simulink model "AmpelkreuzungV4_7"  (R2024b)
settings: Solver=FixedStepAuto  StartTime=0.0  StopTime=450  FixedStep=1  RelTol=1e-3
model workspace (MATLAB code in the model file):
  | function [autos_l1, autos_rg1, autos_2l, autos_2rg, autos_3l, autos_3rg, autos_4, fehler] = generateCars(Auslastung)
  |     if (auslastung == 1)
  |         autos_l1 = round(randn());
  |         autos_rg1 = round(randn());
  |         autos_2l = round(randn());
  |         autos_2rg = round(randn());
  |         autos_3l = round(randn());
  |         autos_3rg = round(randn());
  |         autos_4 = round(randn());
  |     else
  |         fehler = 1;
  |     end
  | 
  |     if (auslastung == 2)
  |         autos_l1 = round(randn());
  |         autos_rg1 = round(4 + 2 * randn());
  |         autos_2l = round(1 + randn());
  |         autos_2rg = round(4 + 2 * randn());
  |         autos_3l = round(randn());
  |         autos_3rg = round(2 + randn());
  |         autos_4 = round(1 + randn());
  |     else
  |         fehler = 1;
  |     end
  | 
  |     if (auslastung == 3)
  |         autos_l1 = round(1.5 + randn());
  |         autos_rg1 = round(7 + 2 * randn());
  |         autos_2l = round(2 + randn());
  |         autos_2rg = round(7 + 2 * randn());
  |         autos_3l = round(2 * randn());
  |         autos_3rg = round(3 + randn());
  |         autos_4 = round(2 + randn());
  |     else
  |         fehler = 1;
  |     end
  | 
  |     if (auslastung == 4)
  |         autos_l1 = round(2.5 + randn());
  |         autos_rg1 = round(13 + 3 * randn());
  |         autos_2l = round(5 + randn());
  |         autos_2rg = round(13 + 3 * randn());
  |         autos_3l = round(2 + randn());
  |         autos_3rg = round(2 + randn());
  |         autos_4 = round(5 + randn());
  |     else
  |         fehler = 1;
  |     end
  | end
(part 2 of 2)

== stateflow chart AmpelkreuzungV4_7/Chart ==
  state Start
    entry:
    rot1_l = 1;
    gelb1_l = 0;
    gruen1_l = 0;
    rot1_rg = 1;
    gelb1_rg = 0;
    gruen1_rg = 0;
    rot2 = 1;
    gelb2 = 0;
    gruen2 = 0;
    rot3_l = 1;
    gelb3_l = 0;
    gruen3_l = 0;
    rot3_rg = 1;
    gelb3_rg = 0;
    gruen3_rg = 0;
    rot4 = 1;
    gelb4 = 0;
    gruen4 = 0;
    rot5 = 1;
    gruen5 = 0;
    rot6 = 1;
    gruen6 = 0;
    rot7 = 1;
    gruen7 = 0;
    rot8 = 1;
    gruen8 = 0;
    timeCounter = 0;
    timer_spuren = [0 0 0 0 0 0 0];
    gesamtZeit = 0;
    %alle_autos = [0 0 0 0 0 0 0; 0 0 0 0 0 0 0];
    spur1 = zeros(1,N/2);
    spur2 = zeros(1,N/2);
    spur3 = zeros(1,N/2);
    spur4 = zeros(1,N/2);
    spur5 = zeros(1,N/2);
    spur6 = zeros(1,N/2);
    spur7 = zeros(1,N/2);
    autos_auf_spur1 = 0;
    autos_auf_spur2 = 0;
    autos_auf_spur3 = 0;
    autos_auf_spur4 = 0;
    autos_auf_spur5 = 0;
    autos_auf_spur6 = 0;
    autos_auf_spur7 = 0;
    counter = [0 0 0 0 0 0 0];
    anz_autos1 = 0;
    anz_autos2 = 0;
    anz_autos3 = 0;
    anz_autos4 = 0;
    anz_autos5 = 0;
    anz_autos6 = 0;
    anz_autos7 = 0;
    wartezeit_spur1_ges = 0;
    wartezeit_spur2_ges = 0;
    wartezeit_spur3_ges = 0;
    wartezeit_spur4_ges = 0;
    wartezeit_spur5_ges = 0;
    wartezeit_spur6_ges = 0;
    wartezeit_spur7_ges = 0;
  state dokumentiere_startzeiten_initialisiere_wartezeiten
    en:
    startzeiten1 = spur1;
    startzeiten2 = spur2;
    startzeiten3 = spur3;
    startzeiten4 = spur4;
    startzeiten5 = spur5;
    startzeiten6 = spur6;
    startzeiten7 = spur7;
    wartezeiten1 = zeros(1, length(startzeiten1));
    wartezeiten2 = zeros(1, length(startzeiten2));
    wartezeiten3 = zeros(1, length(startzeiten3));
    wartezeiten4 = zeros(1, length(startzeiten4));
    wartezeiten5 = zeros(1, length(startzeiten5));
    wartezeiten6 = zeros(1, length(startzeiten6));
    wartezeiten7 = zeros(1, length(startzeiten7));
  state endzeiten_initialisieren
    en:
    endzeiten1 = zeros(1, length(spur1));
    endzeiten2 = zeros(1, length(spur2));
    endzeiten3 = zeros(1, length(spur3));
    endzeiten4 = zeros(1, length(spur4));
    endzeiten5 = zeros(1, length(spur5));
    endzeiten6 = zeros(1, length(spur6));
    endzeiten7 = zeros(1, length(spur7));
  state rg1_ampel2_rotgelb
    entry:
    gelb1_rg = 1;
    gelb2 = 1;
  state l1_rg1_rotgelb
    entry:
    gelb1_l = 1;
    gelb1_rg = 1;
  state rg1_ampel2_gruen
    entry:
    rot1_rg = 0;
    gelb1_rg = 0;
    gruen1_rg = 1;
    rot2 = 0;
    gelb2 = 0;
    gruen2 = 1;
    rot7 = 0;
    gruen7 = 1;
    rot8 = 0;
    gruen8 = 1;
  state l1_rg1_gruen
    entry:
    rot1_l = 0;
    gelb1_l = 0;
    gruen1_l = 1;
    rot1_rg = 0;
    gelb1_rg = 0;
    gruen1_rg = 1;
    rot7 = 0;
    gruen7 = 1;
  state l1_gelb
    entry:
    gelb1_l = 1;
    gruen1_l = 0;
  state l1_rot
    entry:
    rot1_l = 1;
    gelb1_l = 0;
  state Fuss7_rot1
    entry:
    rot7 = 1;
    gruen7 = 0;
  state l1_rot1
    entry:
    rot1_l = 1;
    gelb1_l = 0;
  state rg1_gelb1
    entry:
    gelb1_rg = 1;
    gruen1_rg = 0;
  state ampel2_rotgelb
    entry:
    gelb2 = 1;
  state ampel2_fuss8_gruen
    rot2 = 0;
    gelb2 = 0;
    gruen2 = 1;
    rot8 = 0;
    gruen8 = 1;
  state rg1_rot1
    entry:
    gelb1_rg = 0;
    rot1_rg = 1;
  state Fuss7_rot
    entry:
    rot7 = 1;
    gruen7 = 0;
  state rg1_gelb
    entry:
    gelb1_rg = 1;
    gruen1_rg = 0;
  state rg1_rot
    entry:
    gelb1_rg = 0;
    rot1_rg = 1;
  state rg1_rot5
    entry:
    gelb1_rg = 0;
    rot1_rg = 1;
  state rg1_rot4
    entry:
    gelb1_rg = 0;
    rot1_rg = 1;
  state rg1_rot3
    entry:
    gelb1_rg = 0;
    rot1_rg = 1
  state rg1_rot2
    entry:
    gelb1_rg = 0;
    rot1_rg = 1
  state fuss8_rot1
    entry:
    rot8 = 1;
    gruen8 = 0;
  state fuss8_rot
    entry:
    rot8 = 1;
    gruen8 = 0;
  state ampel2_gelb1
    entry:
    gelb2 = 1;
    gruen2 = 0;
  state ampel2_gelb
    entry:
    gelb2 = 1;
    gruen2 = 0;
  state ampel2_rot
    rot2 = 1;
    gelb2 = 0;
  state ampel2_rot1
    rot2 = 1;
    gelb2 = 0;
  state ampel2_rot2
    rot2 = 1;
    gelb2 = 0;
  state ampel2_rot3
    rot2 = 1;
    gelb2 = 0;
  state rg3_rotgelb
    entry:
    gelb3_rg = 1;
  state rg3_rotgelb1
    entry:
    gelb3_rg = 1;
  state l3_rotgelb_rg3_fuss6_gruen
    entry:
    gelb3_l = 1;
    rot3_rg = 0;
    gelb3_rg = 0;
    gruen3_rg = 1;
    rot6 = 0;
    gruen6 = 1;
  state rg3_fuss6_gruen
    entry:
    rot3_rg = 0;
    gelb3_rg = 0;
    gruen3_rg = 1;
    rot6 = 0;
    gruen6 = 1;
  state ampel4_rotgelb
    entry:
    gelb4 = 1;
  state l3_gruen
    entry:
    rot3_l = 0;
    gelb3_l = 0;
    gruen3_l = 1;
  state l3_gelb
    entry:
    gelb3_l = 1;
    gruen3_l = 0;
  state ampel4_fuss5_gruen
    entry:
    rot4 = 0;
    gelb4 = 0;
    gruen4 = 1;
    rot5 = 0;
    gruen5 = 1;
  state l3_fuss6_rot
    entry:
    rot3_l = 1;
    gelb3_l = 0;
    rot6 = 1;
    gruen6 = 0;
  state l3_fuss6_rot1
    entry:
    rot3_l = 1;
    gelb3_l = 0;
    rot6 = 1;
    gruen6 = 0;
  state fuss6_rot
    entry:
    rot6 = 1;
    gruen6 = 0;
  state rg3_gelb1
    entry:
    gelb3_rg = 1;
    gruen3_rg = 0;
  state rg3_gelb
    entry:
    gelb3_rg = 1;
    gruen3_rg = 0;
  state rg3_rot_ampel4_rotgelb
    entry:
    rot3_rg = 1;
    gelb3_rg = 0;
    gelb4 = 1;
  state rg3_fuss5_rot
    entry:
    rot3_rg = 1;
    gelb3_rg = 0;
    rot5 = 1;
    gruen5 = 0;
  state rg3_rot_ampel4_rotgelb1
    entry:
    rot3_rg = 1;
    gelb3_rg = 0;
    gelb4 = 1;
  state ampel4_fuss5_gruen1
    entry:
    rot4 = 0;
    gelb4 = 0;
    gruen4 = 1;
    rot5 = 0;
    gruen5 = 1;
  state fuss5_rot
    entry:
    rot5 = 1;
    gruen5 = 0;
  state rg3_fuss5_rot1
    entry:
    rot3_rg = 1;
    gelb3_rg = 0;
    rot5 = 1;
    gruen5 = 0;
  state ampel4_gelb
    entry:
    gelb4 = 1;
    gruen4 = 0;
  state ampel4_rot
    entry:
    rot4 = 1;
    gelb4 = 0;
  state ampel4_rot2
    entry:
    rot4 = 1;
    gelb4 = 0;
  (default) -> Start
  Start -> (junction 796) : {zeit_abstand = zeit_abstand_aus_auslastung(auslastung);}
  (junction 796) -> (junction 748) : {alle_autos_neu  = generiere_autos_neu(N, zeit_abstand);}
  (junction 748) -> dokumentiere_startzeiten_initialisiere_wartezeiten : {[spur1, spur2, spur3, spur4, spur5, spur6, spur7] = spuren_aus_autos(alle_autos_neu, N);}
  dokumentiere_startzeiten_initialisiere_wartezeiten -> endzeiten_initialisieren
  endzeiten_initialisieren -> (junction 248)
  (junction 181) -> (junction 248) : {timeCounter = resetTimer()}
  (junction 179) -> (junction 181)
  (junction 248) -> (junction 250) : {alte_counter = counter;}
  (junction 250) -> (junction 442) : after(1,sec)
      | {timeCounter = refresher(timeCounter, 1);}
  (junction 442) -> (junction 757) : {timer_spuren = countOnwards(timer_spuren,1,[1 1 1 1 1 1 1]);}
      |
      | %Linksabbieger1
  (junction 757) -> (junction 15) : {[autos_auf_spur1, spur1] = autos_auf_spur_generieren(spur1, gesamtZeit + timeCounter + 2, autos_auf_spur1);}
  (junction 15) -> (junction 69) [order 1] : [autos_auf_spur1 == 0]
  (junction 15) -> (junction 17) [order 2]
  (junction 69) -> rg1_ampel2_rotgelb
  (junction 17) -> (junction 18) [order 1] : [autos_auf_spur1 > 0]
  (junction 17) -> (junction 19) [order 2]
  (junction 18) -> l1_rg1_rotgelb
  rg1_ampel2_rotgelb -> (junction 755) : after(1,sec)
      | {timeCounter = refresher(timeCounter, 1);}
  l1_rg1_rotgelb -> (junction 444) : after(1,sec)
      | {timeCounter = refresher(timeCounter, 1);}
  (junction 755) -> rg1_ampel2_gruen : {timer_spuren = countOnwards(timer_spuren,1,[1 1 1 1 1 1 1]);}
  (junction 444) -> l1_rg1_gruen : {timer_spuren = countOnwards(timer_spuren,1,[1 1 1 1 1 1 1]);}
  rg1_ampel2_gruen -> (junction 643) : {[autos_auf_spur2, spur2] = autos_auf_spur_generieren(spur2, gesamtZeit + timeCounter, autos_auf_spur2);}
  (junction 643) -> (junction 647) : {[autos_auf_spur3, spur3] = autos_auf_spur_generieren(spur3, gesamtZeit + timeCounter, autos_auf_spur3);}
  l1_rg1_gruen -> (junction 645) : {[autos_auf_spur1, spur1] = autos_auf_spur_generieren(spur1, gesamtZeit + timeCounter, autos_auf_spur1);}
  (junction 645) -> (junction 622) : {[autos_auf_spur2, spur2] = autos_auf_spur_generieren(spur2, gesamtZeit + timeCounter, autos_auf_spur2);}
  (junction 647) -> (junction 641) : {[autos_auf_spur4, spur4] = autos_auf_spur_generieren(spur4, gesamtZeit + timeCounter, autos_auf_spur4);}
  (junction 622) -> (junction 446) : after(7,sec)
      | {timeCounter = refresher(timeCounter, 7);}
  (junction 446) -> l1_gelb : {timer_spuren = countOnwards(timer_spuren,7,[0 0 1 1 1 1 1]);}
  (junction 641) -> (junction 483) : after(25,sec)
      | {timeCounter = refresher(timeCounter, 25);}
  l1_gelb -> (junction 449) : after(3,sec)
      | {timeCounter = refresher(timeCounter, 3);}
  (junction 483) -> Fuss7_rot1 : {timer_spuren = countOnwards(timer_spuren,25,[1 0 0 0 1 1 1]);}
  (junction 449) -> (junction 768) : {[autos_auf_spur1, spur1] = autos_auf_spur_generieren(spur1, gesamtZeit + timeCounter, autos_auf_spur1);}
  (junction 768) -> l1_rot : {timer_spuren = countOnwards(timer_spuren,3,[0 0 1 1 1 1 1]);}
  l1_rot -> (junction 889) : {[anz_autos1, autos_auf_spur1, counter(1), endzeiten1] = generiere_gruenphase(1, 10, autos_auf_spur1, counter(1),  (gesamtZeit + timeCounter -10 ), endzeiten1, startzeiten1);}
  (junction 889) -> (junction 895) : {wartezeiten1 = berechne_wartezeiten(startzeiten1, endzeiten1, alte_counter(1), counter(1), wartezeiten1)}
  (junction 895) -> (junction 891) : {wartezeit_spur1_ges = gesamt_wartezeit_pro_spur(wartezeiten1, wartezeit_spur1_ges, alte_counter(1), counter(1))}
  Fuss7_rot1 -> (junction 485) : after(2,sec)
      | {timeCounter = refresher(timeCounter, 2);}
  (junction 891) -> (junction 893) : {gesamtwartezeit = berechne_gesamtwartezeit(wartezeit_spur1_ges, wartezeit_spur2_ges, wartezeit_spur3_ges, wartezeit_spur4_ges, wartezeit_spur5_ges, wartezeit_spur6_ges, wartezeit_spur7_ges)}
  (junction 485) -> rg1_gelb1 : {timer_spuren = countOnwards(timer_spuren,2,[1 0 0 0 1 1 1]);}
  (junction 893) -> l1_rot1 : {gesamte_autos = berechne_gesamte_autos(counter(1), counter(2), counter(3), counter(4), counter(5), counter(6), counter(7))}
  l1_rot1 -> (junction 451) : after(3,sec)
      | {timeCounter = refresher(timeCounter, 3);}
  rg1_gelb1 -> (junction 772) : after(3,sec)
      | {timeCounter = refresher(timeCounter, 3);}
  (junction 451) -> ampel2_rotgelb : {timer_spuren = countOnwards(timer_spuren,3,[1 0 1 1 1 1 1]);}
  (junction 772) -> (junction 487) : {[autos_auf_spur2, spur2] = autos_auf_spur_generieren(spur2, gesamtZeit + timeCounter, autos_auf_spur2);}
  ampel2_rotgelb -> (junction 464) : after(1,sec)
      | {timeCounter = refresher(timeCounter, 1);}
  (junction 464) -> ampel2_fuss8_gruen : {timer_spuren = countOnwards(timer_spuren,1,[1 0 1 1 1 1 1]);}
  (junction 487) -> rg1_rot1 : {timer_spuren = countOnwards(timer_spuren,3,[1 0 0 0 1 1 1]);}
  ampel2_fuss8_gruen -> (junction 765) : {[autos_auf_spur3, spur3] = autos_auf_spur_generieren(spur3, gesamtZeit + timeCounter, autos_auf_spur3);}
  rg1_rot1 -> (junction 910) : {[anz_autos2, autos_auf_spur2, counter(2), endzeiten2] = generiere_gruenphase(2, 30, autos_auf_spur2, counter(2),  (gesamtZeit + timeCounter -30 ), endzeiten2, startzeiten2);}
  (junction 765) -> (junction 759) : {[autos_auf_spur4, spur4] = autos_auf_spur_generieren(spur4, gesamtZeit + timeCounter, autos_auf_spur4);}
  (junction 759) -> (junction 473) : after(25,sec)
      | {timeCounter = refresher(timeCounter, 25);}
  (junction 473) -> Fuss7_rot : {timer_spuren = countOnwards(timer_spuren,25,[1 0 0 0 1 1 1]);}
  (junction 910) -> (junction 914) : {wartezeiten2 = berechne_wartezeiten(startzeiten2, endzeiten2, alte_counter(2), counter(2), wartezeiten2)}
  Fuss7_rot -> (junction 475) : after(2,sec)
      | {timeCounter = refresher(timeCounter, 2);}
  (junction 914) -> (junction 912) : {wartezeit_spur2_ges = gesamt_wartezeit_pro_spur(wartezeiten2, wartezeit_spur2_ges, alte_counter(2), counter(2))}
  (junction 475) -> rg1_gelb : {timer_spuren = countOnwards(timer_spuren,2,[1 0 0 0 1 1 1]);}
  (junction 912) -> (junction 913) : {gesamtwartezeit = berechne_gesamtwartezeit(wartezeit_spur1_ges, wartezeit_spur2_ges, wartezeit_spur3_ges, wartezeit_spur4_ges, wartezeit_spur5_ges, wartezeit_spur6_ges, wartezeit_spur7_ges)}
  rg1_gelb -> (junction 477) : after(3,sec)
      | {timeCounter = refresher(timeCounter, 3);}
  (junction 477) -> (junction 770) : {[autos_auf_spur2, spur2] = autos_auf_spur_generieren(spur2, gesamtZeit + timeCounter, autos_auf_spur2);}
  (junction 770) -> rg1_rot : {timer_spuren = countOnwards(timer_spuren,3,[1 0 0 0 1 1 1]);}
  (junction 913) -> rg1_rot5 : {gesamte_autos = berechne_gesamte_autos(counter(1), counter(2), counter(3), counter(4), counter(5), counter(6), counter(7))}
  rg1_rot -> (junction 898) : {[anz_autos2, autos_auf_spur2, counter(2), endzeiten2] = generiere_gruenphase(2, 44, autos_auf_spur2, counter(2),  (gesamtZeit + timeCounter - 44 ), endzeiten2, startzeiten2);}
  (junction 898) -> (junction 903) : {wartezeiten2 = berechne_wartezeiten(startzeiten2, endzeiten2, alte_counter(2), counter(2), wartezeiten2)}
  rg1_rot5 -> (junction 71)
  (junction 903) -> (junction 900) : {wartezeit_spur2_ges = gesamt_wartezeit_pro_spur(wartezeiten2, wartezeit_spur2_ges, alte_counter(2), counter(2))}
  (junction 900) -> (junction 902) : {gesamtwartezeit = berechne_gesamtwartezeit(wartezeit_spur1_ges, wartezeit_spur2_ges, wartezeit_spur3_ges, wartezeit_spur4_ges, wartezeit_spur5_ges, wartezeit_spur6_ges, wartezeit_spur7_ges)}
  (junction 902) -> rg1_rot4 : {gesamte_autos = berechne_gesamte_autos(counter(1), counter(2), counter(3), counter(4), counter(5), counter(6), counter(7))}
  rg1_rot4 -> (junction 20)
  (junction 20) -> (junction 19)
  (junction 71) -> (junction 20)
  (junction 19) -> (junction 199)
  (junction 199) -> rg1_rot3 [order 1] : [autos_auf_spur3 <= 2]
  (junction 199) -> (junction 201) [order 2]
  rg1_rot3 -> (junction 498) : after(7,sec)
      | {timeCounter = refresher(timeCounter, 7);}
  (junction 201) -> rg1_rot2 [order 1] : [autos_auf_spur3 > 2]
  (junction 201) -> (junction 203) [order 2]
  rg1_rot2 -> (junction 489) : after(20,sec)
      | {timeCounter = refresher(timeCounter, 20);}
  (junction 498) -> fuss8_rot1 : {timer_spuren = countOnwards(timer_spuren,7,[1 1 0 0 1 1 1]);}
  (junction 489) -> fuss8_rot : {timer_spuren = countOnwards(timer_spuren,20,[1 1 0 0 1 1 1]);}
  fuss8_rot1 -> (junction 500) : after(2,sec)
      | {timeCounter = refresher(timeCounter, 2);}
  fuss8_rot -> (junction 491) : after(2,sec)
      | {timeCounter = refresher(timeCounter, 2);}
  (junction 500) -> ampel2_gelb1 : {timer_spuren = countOnwards(timer_spuren,2,[1 1 0 0 1 1 1]);}
  (junction 491) -> ampel2_gelb : {timer_spuren = countOnwards(timer_spuren,2,[1 1 0 0 1 1 1]);}
  ampel2_gelb1 -> (junction 502) : after(3,sec)
      | {timeCounter = refresher(timeCounter, 3);}
  ampel2_gelb -> (junction 493) : after(3,sec)
      | {timeCounter = refresher(timeCounter, 3);}
  (junction 493) -> (junction 776) : {timer_spuren = countOnwards(timer_spuren,3,[1 1 0 0 1 1 1]);}
  (junction 502) -> (junction 780) : {timer_spuren = countOnwards(timer_spuren,3,[1 1 0 0 1 1 1]);}
  (junction 776) -> (junction 778) : {[autos_auf_spur3, spur3] = autos_auf_spur_generieren(spur3, gesamtZeit + timeCounter, autos_auf_spur3);}
  (junction 780) -> (junction 782) : {[autos_auf_spur3, spur3] = autos_auf_spur_generieren(spur3, gesamtZeit + timeCounter, autos_auf_spur3);}
  (junction 778) -> ampel2_rot : {[autos_auf_spur4, spur4] = autos_auf_spur_generieren(spur4, gesamtZeit + timeCounter, autos_auf_spur4);}
  (junction 782) -> ampel2_rot1 : {[autos_auf_spur4, spur4] = autos_auf_spur_generieren(spur4, gesamtZeit + timeCounter, autos_auf_spur4);}
  ampel2_rot -> (junction 919) : {[anz_autos3, autos_auf_spur3, counter(3), endzeiten3] = generiere_gruenphase(3, 55, autos_auf_spur3, counter(3),  (gesamtZeit + timeCounter -55), endzeiten3, startzeiten3);}
  (junction 919) -> (junction 923) : {wartezeiten3 = berechne_wartezeiten(startzeiten3, endzeiten3, alte_counter(3), counter(3), wartezeiten3)}
  (junction 923) -> (junction 921) : {wartezeit_spur3_ges = gesamt_wartezeit_pro_spur(wartezeiten3, wartezeit_spur3_ges, alte_counter(3), counter(3))}
  ampel2_rot1 -> (junction 946) : {[anz_autos3, autos_auf_spur3, counter(3), endzeiten3] = generiere_gruenphase(3, 42, autos_auf_spur3, counter(3),  (gesamtZeit + timeCounter - 42), endzeiten3, startzeiten3);}
  (junction 921) -> (junction 922) : {gesamtwartezeit = berechne_gesamtwartezeit(wartezeit_spur1_ges, wartezeit_spur2_ges, wartezeit_spur3_ges, wartezeit_spur4_ges, wartezeit_spur5_ges, wartezeit_spur6_ges, wartezeit_spur7_ges)}
  (junction 946) -> (junction 950) : {wartezeiten3 = berechne_wartezeiten(startzeiten3, endzeiten3, alte_counter(3), counter(3), wartezeiten3)}
  (junction 922) -> (junction 750) : {gesamte_autos = berechne_gesamte_autos(counter(1), counter(2), counter(3), counter(4), counter(5), counter(6), counter(7))}
  (junction 950) -> (junction 948) : {wartezeit_spur3_ges = gesamt_wartezeit_pro_spur(wartezeiten3, wartezeit_spur3_ges, alte_counter(3), counter(3))}
  (junction 750) -> (junction 928) : {[anz_autos4, autos_auf_spur4, counter(4), endzeiten4] = generiere_gruenphase(4, 55, autos_auf_spur4, counter(4),  (gesamtZeit + timeCounter -55), endzeiten4, startzeiten4);}
  (junction 948) -> (junction 949) : {gesamtwartezeit = berechne_gesamtwartezeit(wartezeit_spur1_ges, wartezeit_spur2_ges, wartezeit_spur3_ges, wartezeit_spur4_ges, wartezeit_spur5_ges, wartezeit_spur6_ges, wartezeit_spur7_ges)}
  (junction 928) -> (junction 932) : {wartezeiten4 = berechne_wartezeiten(startzeiten4, endzeiten4, alte_counter(4), counter(4), wartezeiten4)}
  (junction 949) -> (junction 656) : {gesamte_autos = berechne_gesamte_autos(counter(1), counter(2), counter(3), counter(4), counter(5), counter(6), counter(7))}
  (junction 932) -> (junction 930) : {wartezeit_spur4_ges = gesamt_wartezeit_pro_spur(wartezeiten4, wartezeit_spur4_ges, alte_counter(4), counter(4))}
  (junction 656) -> (junction 954) : {[anz_autos4, autos_auf_spur4, counter(4), endzeiten4] = generiere_gruenphase(4, 42, autos_auf_spur4, counter(4),  (gesamtZeit + timeCounter -42), endzeiten4, startzeiten4);}
  (junction 954) -> (junction 958) : {wartezeiten4 = berechne_wartezeiten(startzeiten4, endzeiten4, alte_counter(4), counter(4), wartezeiten4)}
  (junction 930) -> (junction 931) : {gesamtwartezeit = berechne_gesamtwartezeit(wartezeit_spur1_ges, wartezeit_spur2_ges, wartezeit_spur3_ges, wartezeit_spur4_ges, wartezeit_spur5_ges, wartezeit_spur6_ges, wartezeit_spur7_ges)}
  (junction 958) -> (junction 956) : {wartezeit_spur4_ges = gesamt_wartezeit_pro_spur(wartezeiten4, wartezeit_spur4_ges, alte_counter(4), counter(4))}
  (junction 931) -> ampel2_rot2 : {gesamte_autos = berechne_gesamte_autos(counter(1), counter(2), counter(3), counter(4), counter(5), counter(6), counter(7))}
  (junction 956) -> (junction 957) : {gesamtwartezeit = berechne_gesamtwartezeit(wartezeit_spur1_ges, wartezeit_spur2_ges, wartezeit_spur3_ges, wartezeit_spur4_ges, wartezeit_spur5_ges, wartezeit_spur6_ges, wartezeit_spur7_ges)}
  (junction 957) -> ampel2_rot3 : {gesamte_autos = berechne_gesamte_autos(counter(1), counter(2), counter(3), counter(4), counter(5), counter(6), counter(7))}
  ampel2_rot2 -> (junction 495) : after(1,sec)
      | {timeCounter = refresher(timeCounter, 1);}
  ampel2_rot3 -> (junction 504) : after(1,sec)
      | {timeCounter = refresher(timeCounter, 1);}
  (junction 495) -> rg3_rotgelb : {timer_spuren = countOnwards(timer_spuren,1,[1 1 1 1 1 1 1]);}
  (junction 504) -> rg3_rotgelb1 : {timer_spuren = countOnwards(timer_spuren,1,[1 1 1 1 1 1 1]);}
  rg3_rotgelb -> (junction 204)
  rg3_rotgelb1 -> (junction 205)
  (junction 204) -> (junction 203)
  (junction 205) -> (junction 204)
  (junction 203) -> (junction 115) : {[autos_auf_spur5, spur5] = autos_auf_spur_generieren(spur5, gesamtZeit + timeCounter, autos_auf_spur5);}
  (junction 115) -> (junction 116) [order 1] : [autos_auf_spur5 == 0]
  (junction 115) -> (junction 117) [order 2]
  (junction 116) -> (junction 526) : after(1,sec)
      | {timeCounter = refresher(timeCounter, 1);}
  (junction 117) -> (junction 118) [order 1] : [autos_auf_spur5 > 0]
  (junction 117) -> (junction 119) [order 2]
  (junction 118) -> l3_rotgelb_rg3_fuss6_gruen
  (junction 526) -> rg3_fuss6_gruen : {timer_spuren = countOnwards(timer_spuren,1,[1 1 1 1 1 1 1]);}
  l3_rotgelb_rg3_fuss6_gruen -> (junction 660) : {[autos_auf_spur6, spur6] = autos_auf_spur_generieren(spur6, gesamtZeit + timeCounter, autos_auf_spur6);}
  rg3_fuss6_gruen -> (junction 671) : {[autos_auf_spur6, spur6] = autos_auf_spur_generieren(spur6, gesamtZeit + timeCounter, autos_auf_spur6);}
  (junction 671) -> (junction 530) : after(4,sec)
      | {timeCounter = refresher(timeCounter, 4);}
  (junction 660) -> (junction 508) : after(1,sec)
      | {timeCounter = refresher(timeCounter, 1);}
  (junction 508) -> l3_gruen : {timer_spuren = countOnwards(timer_spuren,1,[1 1 1 1 1 0 1]);}
  (junction 530) -> ampel4_rotgelb : {timer_spuren = countOnwards(timer_spuren,4,[1 1 1 1 1 0 1]);}
  ampel4_rotgelb -> (junction 532) : after(1,sec)
      | {timeCounter = refresher(timeCounter, 1);}
  l3_gruen -> (junction 512) : after(8,sec)
      | {timeCounter = refresher(timeCounter, 8);}
  (junction 532) -> ampel4_fuss5_gruen : {timer_spuren = countOnwards(timer_spuren,1,[1 1 1 1 1 0 1]);}
  (junction 512) -> l3_gelb : {timer_spuren = countOnwards(timer_spuren,8,[1 1 1 1 0 0 1]);}
  l3_gelb -> (junction 514) : after(3,sec)
      | {timeCounter = refresher(timeCounter, 3);}
  (junction 514) -> (junction 784) : {timer_spuren = countOnwards(timer_spuren,3,[1 1 1 1 0 0 1]);}
  (junction 784) -> l3_fuss6_rot : {[autos_auf_spur5, spur5] = autos_auf_spur_generieren(spur5, gesamtZeit + timeCounter, autos_auf_spur5);}
  ampel4_fuss5_gruen -> (junction 675) : {[autos_auf_spur7, spur7] = autos_auf_spur_generieren(spur7, gesamtZeit + timeCounter, autos_auf_spur7);}
  (junction 675) -> (junction 536) : after(6,sec)
      | {timeCounter = refresher(timeCounter, 6);}
  l3_fuss6_rot -> (junction 962) : {[anz_autos5, autos_auf_spur5, counter(5), endzeiten5] = generiere_gruenphase(5, 11, autos_auf_spur5, counter(5),  (gesamtZeit + timeCounter -11), endzeiten5, startzeiten5);}
  (junction 962) -> (junction 966) : {wartezeiten5 = berechne_wartezeiten(startzeiten5, endzeiten5, alte_counter(5), counter(5), wartezeiten5)}
  (junction 966) -> (junction 964) : {wartezeit_spur5_ges = gesamt_wartezeit_pro_spur(wartezeiten5, wartezeit_spur5_ges, alte_counter(5), counter(5))}
  (junction 964) -> (junction 965) : {gesamtwartezeit = berechne_gesamtwartezeit(wartezeit_spur1_ges, wartezeit_spur2_ges, wartezeit_spur3_ges, wartezeit_spur4_ges, wartezeit_spur5_ges, wartezeit_spur6_ges, wartezeit_spur7_ges)}
  (junction 965) -> l3_fuss6_rot1 : {gesamte_autos = berechne_gesamte_autos(counter(1), counter(2), counter(3), counter(4), counter(5), counter(6), counter(7))}
  (junction 536) -> fuss6_rot : {timer_spuren = countOnwards(timer_spuren,6,[1 1 1 1 1 0 0]);}
  l3_fuss6_rot1 -> (junction 516) : after(2,sec)
      | {timeCounter = refresher(timeCounter, 2);}
  fuss6_rot -> (junction 538) : after(2,sec)
      | {timeCounter = refresher(timeCounter, 2);}
  (junction 516) -> rg3_gelb1 : {timer_spuren = countOnwards(timer_spuren,2,[1 1 1 1 1 0 1]);}
  (junction 538) -> rg3_gelb : {timer_spuren = countOnwards(timer_spuren,2,[1 1 1 1 1 0 0]);}
  rg3_gelb1 -> (junction 518) : after(3,sec)
      | {timeCounter = refresher(timeCounter, 3);}
  rg3_gelb -> (junction 540) : after(3,sec)
      | {timeCounter = refresher(timeCounter, 3);}
  (junction 518) -> (junction 786) : {timer_spuren = countOnwards(timer_spuren,3,[1 1 1 1 1 0 1]);}
  (junction 540) -> (junction 984) : {timer_spuren = countOnwards(timer_spuren,3,[1 1 1 1 1 0 0]);}
  (junction 786) -> rg3_rot_ampel4_rotgelb : {[autos_auf_spur6, spur6] = autos_auf_spur_generieren(spur6, gesamtZeit + timeCounter, autos_auf_spur6);}
  (junction 984) -> rg3_fuss5_rot : {[autos_auf_spur6, spur6] = autos_auf_spur_generieren(spur6, gesamtZeit + timeCounter, autos_auf_spur6);}
  rg3_rot_ampel4_rotgelb -> (junction 970) : {[anz_autos6, autos_auf_spur6, counter(6), endzeiten6] = generiere_gruenphase(6, 17, autos_auf_spur6, counter(6),  (gesamtZeit + timeCounter -17), endzeiten6, startzeiten6);}
  (junction 970) -> (junction 974) : {wartezeiten6 = berechne_wartezeiten(startzeiten6, endzeiten6, alte_counter(6), counter(6), wartezeiten6)}
  rg3_fuss5_rot -> (junction 978) : {[anz_autos6, autos_auf_spur6, counter(6), endzeiten6] = generiere_gruenphase(6, 17, autos_auf_spur6, counter(6),  (gesamtZeit + timeCounter -17), endzeiten6, startzeiten6);}
  (junction 974) -> (junction 972) : {wartezeit_spur6_ges = gesamt_wartezeit_pro_spur(wartezeiten6, wartezeit_spur6_ges, alte_counter(6), counter(6))}
  (junction 972) -> (junction 973) : {gesamtwartezeit = berechne_gesamtwartezeit(wartezeit_spur1_ges, wartezeit_spur2_ges, wartezeit_spur3_ges, wartezeit_spur4_ges, wartezeit_spur5_ges, wartezeit_spur6_ges, wartezeit_spur7_ges)}
  (junction 973) -> rg3_rot_ampel4_rotgelb1 : {gesamte_autos = berechne_gesamte_autos(counter(1), counter(2), counter(3), counter(4), counter(5), counter(6), counter(7))}
  (junction 978) -> (junction 982) : {wartezeiten2 = berechne_wartezeiten(startzeiten2, endzeiten2, alte_counter(2), counter(2), wartezeiten2)}
  (junction 982) -> (junction 980) : {wartezeit_spur2_ges = gesamt_wartezeit_pro_spur(wartezeiten2, wartezeit_spur2_ges, alte_counter(2), counter(2))}
  rg3_rot_ampel4_rotgelb1 -> (junction 520) : after(1,sec)
      | {timeCounter = refresher(timeCounter, 1);}
  (junction 980) -> (junction 981) : {gesamtwartezeit = berechne_gesamtwartezeit(wartezeit_spur1_ges, wartezeit_spur2_ges, wartezeit_spur3_ges, wartezeit_spur4_ges, wartezeit_spur5_ges, wartezeit_spur6_ges, wartezeit_spur7_ges)}
  (junction 520) -> ampel4_fuss5_gruen1 : {timer_spuren = countOnwards(timer_spuren,1,[1 1 1 1 1 1 1]);}
  (junction 981) -> rg3_fuss5_rot1 : {gesamte_autos = berechne_gesamte_autos(counter(1), counter(2), counter(3), counter(4), counter(5), counter(6), counter(7))}
  ampel4_fuss5_gruen1 -> (junction 669) : {[autos_auf_spur7, spur7] = autos_auf_spur_generieren(spur7, gesamtZeit + timeCounter, autos_auf_spur7);}
  (junction 669) -> (junction 524) : after(11,sec)
      | {timeCounter = refresher(timeCounter, 11);}
  (junction 524) -> fuss5_rot : {timer_spuren = countOnwards(timer_spuren,11,[1 1 1 1 1 1 0]);}
  fuss5_rot -> (junction 120)
  rg3_fuss5_rot1 -> (junction 121)
  (junction 120) -> (junction 119)
  (junction 121) -> (junction 120)
  (junction 119) -> (junction 122) : after(2,sec)
      | {timeCounter = refresher(timeCounter, 2);}
  (junction 122) -> ampel4_gelb : {timer_spuren = countOnwards(timer_spuren,2,[1 1 1 1 1 1 0]);}
  ampel4_gelb -> (junction 543) : after(3,sec)
      | {timeCounter = refresher(timeCounter, 3);}
  (junction 543) -> (junction 788) : {timer_spuren = countOnwards(timer_spuren,3,[1 1 1 1 1 1 0]);}
  (junction 788) -> ampel4_rot : {[autos_auf_spur7, spur7] = autos_auf_spur_generieren(spur7, gesamtZeit + timeCounter, autos_auf_spur7);}
  ampel4_rot -> ampel4_rot2 : {[anz_autos7, autos_auf_spur7, counter(7), endzeiten7] = generiere_gruenphase(7, 16, autos_auf_spur7, counter(7),  (gesamtZeit + timeCounter -16), endzeiten7, startzeiten7);}
  ampel4_rot2 -> (junction 545) : after(4,sec)
      | {timeCounter = refresher(timeCounter, 4);}
  (junction 545) -> (junction 395) : {timer_spuren = countOnwards(timer_spuren,4,[1 1 1 1 1 1 1]);}
  (junction 395) -> (junction 812) : {gesamtZeit = gesamtZeit + timeCounter;}
  (junction 812) -> (junction 813) : {disp(startzeiten1)}
  (junction 813) -> (junction 695) : {disp(endzeiten1)}
  (junction 695) -> (junction 834) : {wartezeiten1 = berechne_wartezeiten(startzeiten1, endzeiten1, alte_counter(1), counter(1), wartezeiten1)}
  (junction 834) -> (junction 835) : {wartezeit_spur1_ges = gesamt_wartezeit_pro_spur(wartezeiten1, wartezeit_spur1_ges, alte_counter(1), counter(1))}
  (junction 835) -> (junction 837) : {wartezeiten2 = berechne_wartezeiten(startzeiten2, endzeiten2, alte_counter(2), counter(2), wartezeiten2)}
  (junction 837) -> (junction 839) : {wartezeit_spur2_ges = gesamt_wartezeit_pro_spur(wartezeiten2, wartezeit_spur2_ges, alte_counter(2), counter(2))}
  (junction 839) -> (junction 704) : {wartezeiten3 = berechne_wartezeiten(startzeiten3, endzeiten3, alte_counter(3), counter(3), wartezeiten3)}
  (junction 704) -> (junction 841) : {wartezeit_spur3_ges = gesamt_wartezeit_pro_spur(wartezeiten3, wartezeit_spur3_ges, alte_counter(3), counter(3))}
  (junction 841) -> (junction 706) : {wartezeiten4 = berechne_wartezeiten(startzeiten4, endzeiten4, alte_counter(4), counter(4), wartezeiten4)}
  (junction 706) -> (junction 843) : {wartezeit_spur4_ges = gesamt_wartezeit_pro_spur(wartezeiten4, wartezeit_spur4_ges, alte_counter(4), counter(4))}
  (junction 843) -> (junction 711) : {wartezeiten5 = berechne_wartezeiten(startzeiten5, endzeiten5, alte_counter(5), counter(5), wartezeiten5)}
  (junction 711) -> (junction 845) : {wartezeit_spur5_ges = gesamt_wartezeit_pro_spur(wartezeiten5, wartezeit_spur5_ges, alte_counter(5), counter(5))}
  (junction 845) -> (junction 801) : {wartezeiten6 = berechne_wartezeiten(startzeiten6, endzeiten6, alte_counter(6), counter(6), wartezeiten6)}
  (junction 801) -> (junction 847) : {wartezeit_spur6_ges = gesamt_wartezeit_pro_spur(wartezeiten6, wartezeit_spur6_ges, alte_counter(6), counter(6))}
  (junction 847) -> (junction 803) : {disp(startzeiten7)}
  (junction 803) -> (junction 708) : {disp(endzeiten7)}
  (junction 708) -> (junction 850) : {wartezeiten7 = berechne_wartezeiten(startzeiten7, endzeiten7, alte_counter(7), counter(7), wartezeiten7)}
  (junction 850) -> (junction 866) : {wartezeit_spur7_ges = gesamt_wartezeit_pro_spur(wartezeiten7, wartezeit_spur7_ges, alte_counter(7), counter(7))}
  (junction 866) -> (junction 887) : {gesamtwartezeit = berechne_gesamtwartezeit(wartezeit_spur1_ges, wartezeit_spur2_ges, wartezeit_spur3_ges, wartezeit_spur4_ges, wartezeit_spur5_ges, wartezeit_spur6_ges, wartezeit_spur7_ges)}
  (junction 887) -> (junction 177) : {gesamte_autos = berechne_gesamte_autos(counter(1), counter(2), counter(3), counter(4), counter(5), counter(6), counter(7))}
  (junction 177) -> (junction 179)
  data: autos_neu_fkt function_output; N_fkt function_input; zeit_abstand_fkt function_input; autos_fkt function_input; spur1fkt function_output; spur2fkt function_output; spur3fkt function_output; spur4fkt function_output; spur5fkt function_output; spur6fkt function_output; spur7fkt function_output; N_fkt function_input; spur_autos function_input; timer function_input; autos_auf_spur_fkt function_input; autos_auf_spur_fkt function_output; spur_autos function_output; spur function_input; laenge function_input; autos_auf_spur_u function_input; counter_alt function_input; start_timer_fkt function_input; endzeiten function_input; anz_autos_fkt function_output; autos_auf_spur_fkt function_output; counter_neu_fkt function_output; endzeiten function_output; startzeiten_fkt function_input; auslastung_fkt function_input; zeit_abstand_fkt function_output; time function_input; timeElapsed function_input; spuren function_input; count_spur function_output; timer function_output; timer function_output; startTime function_input; timeElapsed function_input; startzeiten_fkt function_input; endzeiten_fkt function_input; alter_counter_fkt function_input; counter_fkt function_input; wartezeiten_fkt_u function_input; wartezeiten_fkt function_output; wartezeit_fkt function_input; spur_wartezeit_u function_input; counter_alt_fkt function_input; spur_wartezeit_fkt function_output double; counter_fkt function_input; ges_wartezeit1_fkt function_input; ges_wartezeit2_fkt function_input; ges_wartezeit3_fkt function_input; ges_wartezeit4_fkt function_input; ges_wartezeit5_fkt function_input; ges_wartezeit6_fkt function_input; ges_wartezeit7_fkt function_input; gesamtwartezeit_fkt function_output; counter1_fkt function_input; counter2_fkt function_input; counter3_fkt function_input; counter4_fkt function_input; counter5_fkt function_input; counter6_fkt function_input; counter7_fkt function_input; gesamte_autos_fkt function_output; rot1_l output; gelb1_l output; gruen1_l output; rot1_rg output; gelb1_rg output; gruen1_rg output; rot2 output; gelb2 output; gruen2 output; rot3_l output; gelb3_l output; gruen3_l output; rot3_rg output; gelb3_rg output; gruen3_rg output; rot4 output; gelb4 output; gruen4 output; rot5 output; gruen5 output; rot6 output; gruen6 output; rot7 output; gruen7 output; rot8 output; gruen8 output; timeCounter output; gesamtZeit output; timer_spuren local; anz_autos1 local; anz_autos2 local; anz_autos3 local; anz_autos4 local; anz_autos5 local; anz_autos6 local; anz_autos7 local; alte_counter local; counter local; endzeiten1 local; endzeiten2 local; endzeiten3 local; endzeiten4 local; endzeiten5 local; endzeiten6 local; endzeiten7 local; spur1 local; spur2 local; spur3 local; spur4 local; spur5 local; spur6 local; spur7 local; startzeiten7 local; wartezeiten1 local; startzeiten1 local; startzeiten2 local; startzeiten3 local; startzeiten4 local; startzeiten5 local; startzeiten6 local; wartezeiten2 local; wartezeiten3 local; wartezeiten4 local; wartezeiten5 local; wartezeiten6 local; wartezeiten7 local; autos_auf_spur2 output; autos_auf_spur3 output; autos_auf_spur4 output; autos_auf_spur5 output; autos_auf_spur6 output; autos_auf_spur7 output; autos_auf_spur1 output; alle_autos_neu local; N constant double =600; auslastung input; zeit_abstand local; wartezeit_spur6_ges local; wartezeit_spur1_ges local; wartezeit_spur2_ges local; wartezeit_spur5_ges local; wartezeit_spur3_ges local; wartezeit_spur4_ges local; wartezeit_spur7_ges local; gesamtwartezeit output; gesamte_autos output
  function autos_neu_fkt = generiere_autos_neu(N_fkt, zeit_abstand_fkt):
    | function autos_neu_fkt = generiere_autos_neu(N_fkt, zeit_abstand_fkt)
    |     zeiten_fkt = zeros(1,N_fkt); %Platzhalter für Spawnzeiten
    |     for i=1:N
    |         zeiten_fkt(i) = zeit_abstand_fkt * i + randn();
    |         if zeiten_fkt(i) < 0
    |             zeiten_fkt(i) = 0
    |         end
    |     end
    | 	
    |     switch (zeit_abstand_fkt)
    |         case 10
    |             
    |         case 2.5
    | 
    |         case 1.1
    | 
    |         case 0.7
    | 
    |         case 0.6
    |     end
    |     wahrscheinlichkeiten = [0.06, 0.32, 0.07, 0.25, 0.12, 0.10, 0.13];
    |     spuren_werte = [1, 2, 3, 4, 5, 6, 7]; % Die entsprechenden Werte
    | 
    |     kumulative_wahrscheinlichkeiten = cumsum(wahrscheinlichkeiten);
    | 
    |     zufaellige_nummer = rand(1, N_fkt);
    |     spuren = zeros(1, N_fkt); % Platzhalter für die Spuren
    | 
    |     % Werte basierend auf Wahrscheinlichkeiten zuweisen
    |     for i = 1:N_fkt
    |         spuren(i) = spuren_werte(find(zufaellige_nummer(i) <= kumulative_wahrscheinlichkeiten, 1));
    |     end
    | 
    |     zeiten_fkt = sort(zeiten_fkt);
    | 
    |     autos_neu_fkt = [spuren; zeiten_fkt]
    | end
  function [spur1fkt, spur2fkt, spur3fkt, spur4fkt, spur5fkt, spur6fkt, spur7fkt] = spuren_aus_autos(autos_fkt, N_fkt):
    | function [spur1fkt, spur2fkt, spur3fkt, spur4fkt, spur5fkt, spur6fkt, spur7fkt] = spuren_aus_autos(autos_fkt, N_fkt)
    |     counter1 = 1; counter2 = 1; counter3 = 1; counter4 = 1; counter5 = 1; counter6 = 1; counter7 = 1;
    |     spur1fkt = zeros(1,N_fkt/2);
    |     spur2fkt = zeros(1,N_fkt/2);
    |     spur3fkt = zeros(1,N_fkt/2);
    |     spur4fkt = zeros(1,N_fkt/2);
    |     spur5fkt = zeros(1,N_fkt/2);
    |     spur6fkt = zeros(1,N_fkt/2);
    |     spur7fkt = zeros(1,N_fkt/2);
    |     for i = 1:length(autos_fkt)
    |         switch(autos_fkt(1,i))
    |             case 1
    |                 %spur1fkt
    |                 %spur1fkt(counter1)
    |                 %autos_fkt
    |                 %autos_fkt(2,i)
    |                 spur1fkt(counter1) = autos_fkt(2,i);
    |                 counter1 = counter1 + 1;
    |             case 2
    |                 %spur2fkt
    |                 %spur2fkt(counter2)
    |                 %autos_fkt
    |                 %autos_fkt(2,i)
    |                 spur2fkt(counter2) = autos_fkt(2,i);
    |                 counter2 = counter2 + 1;
    |             case 3
    |                 spur3fkt(counter3) = autos_fkt(2,i);
    |                 counter3 = counter3 + 1;
    |             case 4
    |                 spur4fkt(counter4) = autos_fkt(2,i);
    |                 counter4 = counter4 + 1;
    |             case 5
    |                 spur5fkt(counter5) = autos_fkt(2,i);
    |                 counter5 = counter5 + 1;
    |             case 6
    |                 spur6fkt(counter6) = autos_fkt(2,i);
    |                 counter6 = counter6 + 1;
    |             case 7
    |                 spur7fkt(counter7) = autos_fkt(2,i);
    |                 counter7 = counter7 + 1;
    |             otherwise
    |                 disp('error!');
    |         end
    |     end
    |     spur1fkt
    |     spur2fkt
    |     spur3fkt
    |     spur4fkt
    |     spur5fkt
    |     spur6fkt
    |     spur7fkt
    | 
    | end
  function [autos_auf_spur_fkt, spur_autos] = autos_auf_spur_generieren(spur_autos, timer, autos_auf_spur_fkt):
    | function [autos_auf_spur_fkt, spur_autos] = autos_auf_spur_generieren(spur_autos, timer, autos_auf_spur_fkt)
    |     for i = 1:length(spur_autos)
    |         if (spur_autos(i) < timer && spur_autos(i) ~= 0)
    |             autos_auf_spur_fkt = autos_auf_spur_fkt + 1;
    |             spur_autos(i) = 0;
    |         end
    |     end
    | end
  function [anz_autos_fkt, autos_auf_spur_fkt, counter_neu_fkt, endzeiten] = generiere_gruenphase(spur, laenge, autos_auf_spur_u, counter_alt, start_timer_fkt, endzeiten, startzeiten_fkt):
    | function [anz_autos_fkt, autos_auf_spur_fkt, counter_neu_fkt, endzeiten] = generiere_gruenphase(spur, laenge, autos_auf_spur_u, counter_alt, start_timer_fkt, endzeiten, startzeiten_fkt) 
    |     if (spur == 2 || spur == 4)  
    |         if laenge < 8.9
    |             anz_autos_fkt = round(0.314739 * power(laenge, 1.2629099));
    |             for i = 1:min([anz_autos_fkt,autos_auf_spur_u])
    |                 endzeiten(counter_alt + i) = start_timer_fkt + nthroot((i / 0.314739), 1.2629099);
    |                 if endzeiten(counter_alt + i) < startzeiten_fkt(counter_alt + i)
    |                     endzeiten(counter_alt + i) = startzeiten_fkt(counter_alt + i);
    |                 end
    |                 if (counter_alt + i) > 1
    |                     if endzeiten(counter_alt + i) < (endzeiten(counter_alt + i - 1) + 0.7)
    |                         endzeiten(counter_alt + i) = endzeiten(counter_alt + i - 1) + 0.7;
    |                     end
    |                 end
    |                 if (endzeiten(counter_alt + i) > start_timer_fkt + laenge)
    |                     endzeiten(counter_alt + i) = 0;
    |                     anz_autos_fkt = anz_autos_fkt - (min(anz_autos_fkt, autos_auf_spur_u) - i + 1);
    |                     break
    |                 end
    |             end
    | 
    |         elseif laenge >= 8.9
    |             anz_autos_fkt = round((laenge - 8.9) / 1.4 + 5);
    |             for i = 1:min([anz_autos_fkt,autos_auf_spur_u])
    |                 if i <= 5
    |                     endzeiten(counter_alt + i) = start_timer_fkt + nthroot((i / 0.314739), 1.2629099);
    |                 else
    |                     endzeiten(counter_alt + i) = start_timer_fkt + 8.9 + (i - 5) * 1.5;
    |                 end             
    |                 if endzeiten(counter_alt + i) < startzeiten_fkt(counter_alt + i)
    |                     endzeiten(counter_alt + i) = startzeiten_fkt(counter_alt + i);
    |                 end
    |                 if (counter_alt + i) > 1
    |                     if endzeiten(counter_alt + i) < (endzeiten(counter_alt + i - 1) + 0.7)
    |                         endzeiten(counter_alt + i) = endzeiten(counter_alt + i - 1) + 0.7;
    |                     end
    |                 end
    |                 if (endzeiten(counter_alt + i) > start_timer_fkt + laenge)
    |                     endzeiten(counter_alt + i) = 0;
    |                     anz_autos_fkt = anz_autos_fkt - (min(anz_autos_fkt, autos_auf_spur_u) - i + 1);
    |                     break
    |                 end                   
    |             end
    |         end
    |         
    |     elseif (spur == 1 || spur == 3 || spur == 5 || spur == 6 || spur == 7)
    |         if laenge < 8.3
    |             anz_autos_fkt = round(0.3507674 * power(laenge, 1.2576509));
    |             for i = 1:min([anz_autos_fkt,autos_auf_spur_u])
    |                 endzeiten(counter_alt + i) = start_timer_fkt + nthroot((i / 0.3507674), 1.2576509);
    |                 if endzeiten(counter_alt + i) < startzeiten_fkt(counter_alt + i)
    |                     endzeiten(counter_alt + i) = startzeiten_fkt(counter_alt + i);
    |                 end
    |                 if (counter_alt + i) > 1
    |                     if endzeiten(counter_alt + i) < (endzeiten(counter_alt + i - 1) + 0.9)
    |                         endzeiten(counter_alt + i) = endzeiten(counter_alt + i - 1) + 0.9;
    |                     end
    |                 end
    |                 if (endzeiten(counter_alt + i) > start_timer_fkt + laenge)
    |                     endzeiten(counter_alt + i) = 0;
    |                     anz_autos_fkt = anz_autos_fkt - (min(anz_autos_fkt, autos_auf_spur_u) - i + 1);
    |                     break
    |                 end
    |             end
    | 
    |         elseif laenge >= 8.3
    |             anz_autos_fkt = round((laenge - 8.3) / 1.4 + 5);
    |             for i = 1:min([anz_autos_fkt,autos_auf_spur_u])
    |                 if i<= 5
    |                     endzeiten(counter_alt + i) = start_timer_fkt + nthroot((i / 0.3507674), 1.2576509);
    |                 else
    |                     endzeiten(counter_alt + i) = start_timer_fkt + 8.3 +(i - 5) * 1.4;
    |                 end
    |                 if endzeiten(counter_alt + i) < startzeiten_fkt(counter_alt + i)
    |                     endzeiten(counter_alt + i) = startzeiten_fkt(counter_alt + i);
    |                 end
    |                 if (counter_alt + i) > 1
    |                     if endzeiten(counter_alt + i) < (endzeiten(counter_alt + i - 1) + 0.7)
    |                         endzeiten(counter_alt + i) = endzeiten(counter_alt + i - 1) + 0.7;
    |                     end
    |                 end
    |                 if (endzeiten(counter_alt + i) > start_timer_fkt + laenge)
    |                     endzeiten(counter_alt + i) = 0;
    |                     anz_autos_fkt = anz_autos_fkt - (min(anz_autos_fkt, autos_auf_spur_u) - i + 1);
    |                     break
    |                 end
    |             end
    |         end        
    |     end
    | 
    |     autos_auf_spur_fkt = autos_auf_spur_u - anz_autos_fkt
    |     if autos_auf_spur_fkt < 0
    |         autos_auf_spur_fkt = 0
    |     end
    |     counter_neu_fkt = counter_alt + autos_auf_spur_u - autos_auf_spur_fkt
    |     if counter_neu_fkt < counter_alt
    |         counter_neu_fkt = counter_alt
    |     end
    | end
  function zeit_abstand_fkt = zeit_abstand_aus_auslastung(auslastung_fkt):
    | function zeit_abstand_fkt = zeit_abstand_aus_auslastung(auslastung_fkt)
    |     switch (auslastung_fkt)
    |         case 1
    |             zeit_abstand_fkt = 10
    |         case 2
    |             zeit_abstand_fkt = 2.5
    |         case 3
    |             zeit_abstand_fkt = 1.1
    |         case 4
    |             zeit_abstand_fkt = 0.7
    |         case 5
    |             zeit_abstand_fkt = 0.6
    |         otherwise
    |             zeit_abstand_fkt = -1000
    |     end
    | end
  function count_spur = countOnwards(time, timeElapsed, spuren):
    | function count_spur = countOnwards(time, timeElapsed, spuren)
    |     count_spur = time;
    |     i = 1;
    |     for i = 1 : length(time)
    |         if spuren(i) == 1
    |             count_spur(i) = count_spur(i) + timeElapsed;
    |         end
    |     end
    | end
  function timer = resetTimer:
    | function timer = resetTimer()
    |     timer = 0;
    | end
  function timer = refresher(startTime, timeElapsed):
    | function timer = refresher(startTime, timeElapsed)
    |     timer = startTime + timeElapsed;
    | end
  function wartezeiten_fkt = berechne_wartezeiten(startzeiten_fkt, endzeiten_fkt, alter_counter_fkt, counter_fkt, wartezeiten_fkt_u):
    | function wartezeiten_fkt = berechne_wartezeiten(startzeiten_fkt, endzeiten_fkt, alter_counter_fkt, counter_fkt, wartezeiten_fkt_u)
    |     wartezeiten_fkt = wartezeiten_fkt_u;
    |     for i = (alter_counter_fkt + 1):counter_fkt
    |         wartezeiten_fkt(i) = endzeiten_fkt(i) - startzeiten_fkt(i);
    |     end
    | end
  function spur_wartezeit_fkt = gesamt_wartezeit_pro_spur(wartezeit_fkt, spur_wartezeit_u, counter_alt_fkt, counter_fkt):
    | function spur_wartezeit_fkt = gesamt_wartezeit_pro_spur(wartezeit_fkt, spur_wartezeit_u, counter_alt_fkt, counter_fkt)
    |     spur_wartezeit_fkt = spur_wartezeit_u;
    |     for i = (1 + counter_alt_fkt:counter_fkt)
    |         spur_wartezeit_fkt = spur_wartezeit_fkt + wartezeit_fkt(i)
    |     end
    | end
    | 
    | %Variablen: wartezeit_fkt: Vektor mit Wartezeiten, spur_wartezeit_u:
    | %Gesamt-Wartezeit auf der Spur bis zu dem Zeitpunkt
  function gesamtwartezeit_fkt = berechne_gesamtwartezeit(ges_wartezeit1_fkt, ges_wartezeit2_fkt, ges_wartezeit3_fkt, ges_wartezeit4_fkt, ges_wartezeit5_fkt, ges_wartezeit6_fkt, ges_wartezeit7_fkt):
    | function gesamtwartezeit_fkt = berechne_gesamtwartezeit(ges_wartezeit1_fkt, ges_wartezeit2_fkt, ges_wartezeit3_fkt, ges_wartezeit4_fkt, ges_wartezeit5_fkt, ges_wartezeit6_fkt, ges_wartezeit7_fkt)
    |     gesamtwartezeit_fkt = ges_wartezeit1_fkt + ges_wartezeit2_fkt + ges_wartezeit3_fkt + ges_wartezeit4_fkt + ges_wartezeit5_fkt + ges_wartezeit6_fkt + ges_wartezeit7_fkt;
    | end
  function gesamte_autos_fkt = berechne_gesamte_autos(counter1_fkt, counter2_fkt, counter3_fkt, counter4_fkt, counter5_fkt, counter6_fkt, counter7_fkt):
    | function gesamte_autos_fkt = berechne_gesamte_autos(counter1_fkt, counter2_fkt, counter3_fkt, counter4_fkt, counter5_fkt, counter6_fkt, counter7_fkt)
    |     gesamtwartezeit_fkt = counter1_fkt + counter2_fkt + counter3_fkt + counter4_fkt + counter5_fkt + counter6_fkt + counter7_fkt;
    | end
